simulink model "estimation"  (R2023a)
settings: Solver=ode4  StartTime=0.0  StopTime=10.0  FixedStep=dt  RelTol=1e-3
undefined symbols (not defined in the file or in its folder): dt, gnc, plant, UKF
libraries: aerolibutil x2
settings Model: Creator=hugobuurmeijer  LastModifiedBy=ndelurgio

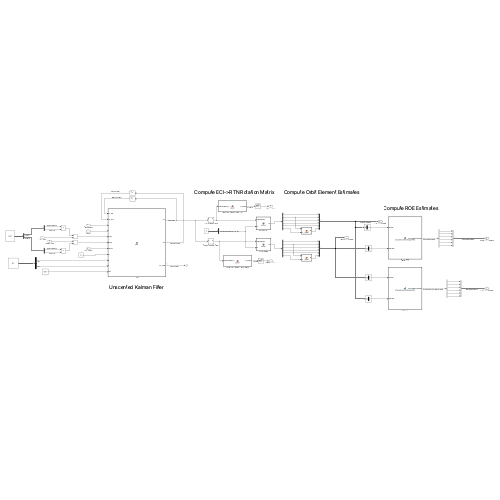
[thumbnail: Simulink's stored preview of the top-level diagram]
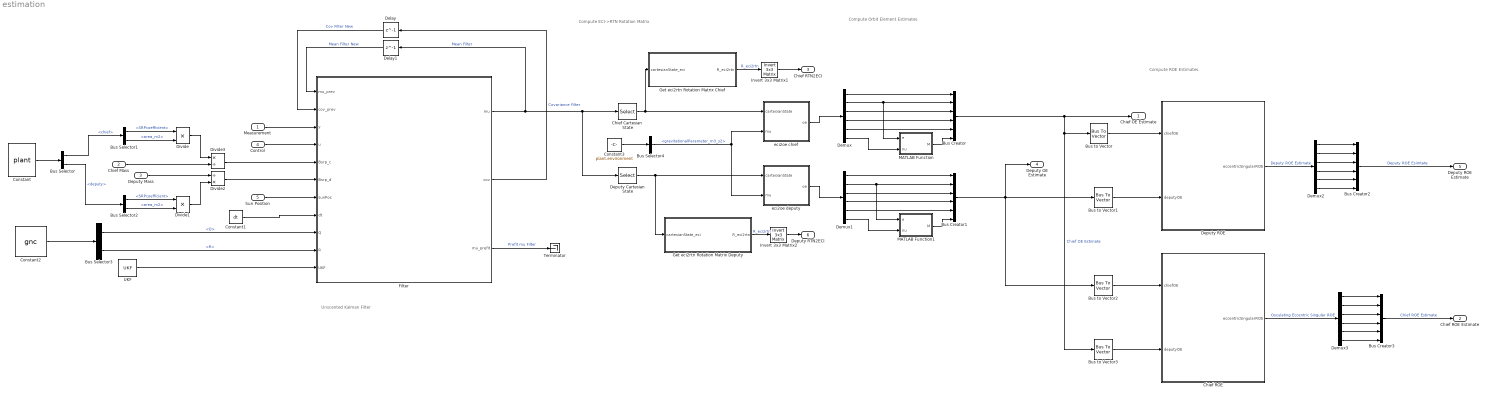
== system estimation ==
  note: Unscented Kalman Filter
  note: Compute Orbit Element Estimates
  note: Compute ROE Estimates
  note: Compute ECI->RTN Rotation Matrix
  Measurement : Inport  PortDimensions=18
  Chief Mass : Inport  Port=2
  Deputy Mass : Inport  Port=3
  Control : Inport  Port=4  PortDimensions=6
  Sun Position : Inport  Port=5  PortDimensions=3
  Bus Creator : BusCreator  Inputs=6  OutDataTypeStr=Bus: osculatingOrbitElements
  Bus Creator1 : BusCreator  Inputs=6  OutDataTypeStr=Bus: osculatingOrbitElements
  Bus Creator2 : BusCreator  Inputs=6  OutDataTypeStr=Bus: eccentricSingularROE
  Bus Creator3 : BusCreator  Inputs=6  OutDataTypeStr=Bus: eccentricSingularROE
  Bus Selector : BusSelector  OutputSignals=chief,deputy
  Bus Selector1 : BusSelector  OutputSignals=properties.SRPcoefficient,properties.area_m2
  Bus Selector2 : BusSelector  OutputSignals=properties.SRPcoefficient,properties.area_m2
  Bus Selector3 : BusSelector  OutputSignals=navigation.Q,navigation.R
  Bus Selector4 : BusSelector  OutputSignals=earthProperties.gravitationalParameter_m3_s2
  Bus to Vector{,1..3} (4 alike) : BusToVector
  Chief Cartesian State : Selector  InputPortWidth=24  IndexOptions=Index vector (dialog)  Indices=1:6  OutputSizes=1
  Chief ROE : MATLAB Function  TreatAsAtomicUnit=on
  Constant : Constant  Value=plant  OutDataTypeStr=Bus: plantBus
  Constant1 : Constant  Value=dt
  Constant2 : Constant  Value=gnc  OutDataTypeStr=Bus: gncBus
  Constant3 : Constant  Value=plant.environment  OutDataTypeStr=Bus: environment
  Delay : Delay  DelayLength=1  InitialCondition=gnc.navigation.covarianceInit
  Delay1 : Delay  DelayLength=1  InitialCondition=gnc.navigation.stateInit
  Demux{,1..3} (4 alike) : Demux  Outputs=6
  Deputy Cartesian State : Selector  InputPortWidth=24  IndexOptions=Index vector (dialog)  Indices=7:12  OutputSizes=1
  Deputy ROE : MATLAB Function  TreatAsAtomicUnit=on
  Divide : Product  Inputs=**
  Divide1 : Product  Inputs=**
  Divide2 : Product  Inputs=/*
  Divide3 : Product  Inputs=*/
  Filter : MATLAB Function  TreatAsAtomicUnit=on
  Get eci2rtn Rotation Matrix Chief : MATLAB Function  TreatAsAtomicUnit=on
  Get eci2rtn Rotation Matrix Deputy : MATLAB Function  TreatAsAtomicUnit=on
  Invert 3x3 Matrix1 : aerolibutil/Invert  3x3 Matrix
  Invert 3x3 Matrix2 : aerolibutil/Invert  3x3 Matrix
  MATLAB Function : MATLAB Function  TreatAsAtomicUnit=on
  MATLAB Function1 : MATLAB Function  TreatAsAtomicUnit=on
  Terminator : Terminator
  UKF : Constant  Value=UKF
  eci2oe chief : MATLAB Function  TreatAsAtomicUnit=on
  eci2oe deputy : MATLAB Function  TreatAsAtomicUnit=on
  Chief OE Estimate : Outport  OutDataTypeStr=Bus: osculatingOrbitElements
  Chief ROE Estimate : Outport  Port=2  OutDataTypeStr=Bus: eccentricSingularROE
  Chief RTN2ECI : Outport  Port=3
  Deputy OE Estimate : Outport  Port=4  OutDataTypeStr=Bus: osculatingOrbitElements
  Deputy ROE Estimate : Outport  Port=5  OutDataTypeStr=Bus: eccentricSingularROE
  Deputy RTN2ECI : Outport  Port=6
  wires:
  Filter/1(mu) -> Deputy Cartesian State/1, Chief Cartesian State/1, Delay1/1  "Mean Filter"
  Filter/2(cov) -> Delay/1  "Covariance Filter"
  Delay/1 -> Filter/2(cov_prev)  "Cov Filter New"
  Delay1/1 -> Filter/1(mu_prev)  "Mean Filter New"
  Measurement/1 -> Filter/3(y)
  Control/1 -> Filter/4(u)
  Constant/1 -> Bus Selector/1
  Bus Selector/1 -> Bus Selector1/1  "<chief>"
  Bus Selector/2 -> Bus Selector2/1  "<deputy>"
  Bus Selector1/2 -> Divide/2  "<area_m2>"
  Bus Selector1/1 -> Divide/1  "<SRPcoefficient>"
  Bus Selector2/2 -> Divide1/2  "<area_m2>"
  Bus Selector2/1 -> Divide1/1  "<SRPcoefficient>"
  Divide1/1 -> Divide2/2
  Deputy Mass/1 -> Divide2/1
  Divide/1 -> Divide3/1
  Chief Mass/1 -> Divide3/2
  Divide3/1 -> Filter/5(Bsrp_c)
  Divide2/1 -> Filter/6(Bsrp_d)
  Sun Position/1 -> Filter/7(sunPos)
  Constant1/1 -> Filter/8(dt)
  Constant2/1 -> Bus Selector3/1
  Bus Selector3/1 -> Filter/9(Q)  "<Q>"
  Bus Selector3/2 -> Filter/10(R)  "<R>"
  Filter/3(mu_prefit) -> Terminator/1  "Prefit mu Filter"
  UKF/1 -> Filter/11(UKF)
  Chief Cartesian State/1 -> eci2oe chief/1(cartesianState), Get eci2rtn Rotation Matrix Chief/1(cartesianState_eci)
  Deputy Cartesian State/1 -> eci2oe deputy/1(cartesianState), Get eci2rtn Rotation Matrix Deputy/1(cartesianState_eci)
  Constant3/1 -> Bus Selector4/1
  Bus Selector4/1 -> eci2oe deputy/2(mu), eci2oe chief/2(mu)  "<gravitationalParameter_m3_s2>"
  eci2oe chief/1(oe) -> Demux/1
  Get eci2rtn Rotation Matrix Chief/1(R_eci2rtn) -> Invert 3x3 Matrix1/1  "R_eci2rtn"
  Get eci2rtn Rotation Matrix Deputy/1(R_eci2rtn) -> Invert 3x3 Matrix2/1  "R_eci2rtn"
  Demux/1 -> Bus Creator/1
  Demux/2 -> MATLAB Function/1(e), Bus Creator/2
  Demux/3 -> Bus Creator/3
  Demux/4 -> Bus Creator/4
  Demux/5 -> Bus Creator/5
  Demux/6 -> MATLAB Function/2(nu)
  Bus Creator/1 -> Chief OE Estimate/1, Bus to Vector3/1, Bus to Vector/1  "Chief OE Estimate"
  Demux1/5 -> Bus Creator1/5
  Bus Creator1/1 -> Deputy OE Estimate/1, Bus to Vector2/1, Bus to Vector1/1
  eci2oe deputy/1(oe) -> Demux1/1
  Demux1/4 -> Bus Creator1/4
  Demux1/3 -> Bus Creator1/3
  Demux1/2 -> MATLAB Function1/1(e), Bus Creator1/2
  Demux1/1 -> Bus Creator1/1
  Demux1/6 -> MATLAB Function1/2(nu)
  Demux2/6 -> Bus Creator2/6
  Demux2/1 -> Bus Creator2/1
  Bus Creator2/1 -> Deputy ROE Estimate/1  "Deputy ROE Esimtate"
  Demux2/5 -> Bus Creator2/5
  Demux2/2 -> Bus Creator2/2
  Demux2/4 -> Bus Creator2/4
  Demux2/3 -> Bus Creator2/3
  Deputy ROE/1(eccentricSingularROE) -> Demux2/1  "Deputy ROE Estimate"
  Demux3/5 -> Bus Creator3/5
  Demux3/4 -> Bus Creator3/4
  Demux3/1 -> Bus Creator3/1
  Demux3/3 -> Bus Creator3/3
  Demux3/6 -> Bus Creator3/6
  Demux3/2 -> Bus Creator3/2
  Bus Creator3/1 -> Chief ROE Estimate/1  "Chief ROE Estimate"
  Chief ROE/1(eccentricSingularROE) -> Demux3/1  "Osculating Eccentric Singular ROE"
  Invert 3x3 Matrix1/1 -> Chief RTN2ECI/1
  Invert 3x3 Matrix2/1 -> Deputy RTN2ECI/1
  MATLAB Function/1(M) -> Bus Creator/6
  MATLAB Function1/1(M) -> Bus Creator1/6
  Bus to Vector/1 -> Deputy ROE/1(chiefOE)
  Bus to Vector1/1 -> Deputy ROE/2(deputyOE)
  Bus to Vector2/1 -> Chief ROE/1(chiefOE)
  Bus to Vector3/1 -> Chief ROE/2(deputyOE)

== matlab function estimation/eci2oe deputy ==
  data: cartesianState input; oe output; mu input
function oe = eci2oe(cartesianState,mu)
[oe,~,~,~] = eci2oe( cartesianState , mu );
end

== matlab function estimation/Filter ==
  data: mu_prev input; cov_prev input; y input; u input; mu output; Bsrp_c input; Bsrp_d input; sunPos input; dt input; Q input; R input; cov output; mu_prefit output; UKF input
function [mu,cov,mu_prefit] = filter(mu_prev,cov_prev, y, u, Bsrp_c, Bsrp_d, sunPos, dt, Q, R, UKF)

if UKF
    [mu,cov,mu_prefit] = ukf(mu_prev,cov_prev, y, u, Bsrp_c, Bsrp_d, sunPos, dt, Q, R);
else
    [mu,cov,mu_prefit] = ekf(mu_prev,cov_prev, y, u, Bsrp_c, Bsrp_d, sunPos, dt, Q, R);
end

== matlab function estimation/eci2oe chief ==
  data: cartesianState input; oe output; mu input
function oe = eci2oe(cartesianState,mu)
[oe,~,~,~] = eci2oe( cartesianState , mu );
end

== matlab function estimation/Deputy ROE ==
  data: chiefOE input; eccentricSingularROE output; deputyOE input
function eccentricSingularROE = computeEccentricSingularROE(chiefOE, deputyOE)

eccentricSingularROE = computeEccentricSingularROE(chiefOE, deputyOE);

end

== matlab function estimation/Chief ROE ==
  data: chiefOE input; eccentricSingularROE output; deputyOE input
function eccentricSingularROE = computeEccentricSingularROE(chiefOE, deputyOE)

eccentricSingularROE = computeEccentricSingularROE(chiefOE, deputyOE);

end

== matlab function estimation/Get eci2rtn Rotation Matrix Chief ==
  data: cartesianState_eci input; R_eci2rtn output
function R_eci2rtn  = eci2rtn(cartesianState_eci)

[~, R_eci2rtn] = eci2rtn(cartesianState_eci);

end

== matlab function estimation/Get eci2rtn Rotation Matrix Deputy ==
  data: cartesianState_eci input; R_eci2rtn output
function R_eci2rtn  = eci2rtn(cartesianState_eci)

[~, R_eci2rtn] = eci2rtn(cartesianState_eci);

end

== matlab function estimation/MATLAB Function ==
  data: e input; M output; nu input
function M = nu2M(e,nu)
M = nu2M(nu,e);
end

== matlab function estimation/MATLAB Function1 ==
  data: e input; M output; nu input
function M = nu2M(e,nu)
M = nu2M(nu,e);
end
